simulink model "processCamera"  (R2014b)
settings: Solver=FixedStepDiscrete  StartTime=0.0  StopTime=inf  RelTol=1e-3
settings Model: DataDictionary=hostData.sldd  Creator=scastro  LastModifiedBy=gsalhotr
settings DataIOCC: SaveOutput=off  SaveTime=off

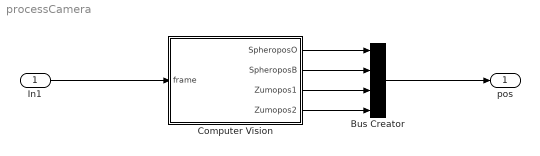
== system processCamera ==
  In1 : Inport
  Bus Creator : BusCreator  OutDataTypeStr=Bus: PositionBus
  Computer Vision : MATLAB Function  TreatAsAtomicUnit=on
  pos : Outport  OutDataTypeStr=Bus: PositionBus
  wires:
  Bus Creator/1 -> pos/1
  In1/1 -> Computer Vision/1(frame)
  Computer Vision/1(SpheroposO) -> Bus Creator/1
  Computer Vision/2(SpheroposB) -> Bus Creator/2
  Computer Vision/3(Zumopos1) -> Bus Creator/3
  Computer Vision/4(Zumopos2) -> Bus Creator/4

== matlab function processCamera/Computer Vision ==
  data: SpheroposO output; SpheroposB output; Zumopos1 output; Zumopos2 output; frame input single size=[480,640,3]
function [SpheroposO, SpheroposB, Zumopos1, Zumopos2] = fcn(frame)
%#codegen

coder.extrinsic('trackTwoMinions')

Zumopos1 = single([0; 0]);
Zumopos2 = single([0; 0]);
SpheroposO = [0; 0];
SpheroposB = [0; 0];
Zumopos = zeros(2, 'single');


[Zumopos, SpheroposO, SpheroposB] = trackTwoMinions(frame, 0);

Zumopos1 = Zumopos(1, :)';
Zumopos2 = Zumopos(2, :)';
